simulink model "pdcm"  (R2019b)
settings: Solver=FixedStepAuto  StartTime=0.0  StopTime=10.0  FixedStep=0.1  RelTol=1e-3
settings Model: Creator=ADEMATO1  LastModifiedBy=EMORAI12
settings SolverCC: PositivePriorityOrder=on  AutoInsertRateTranBlk=on  InsertRTBMode=Always

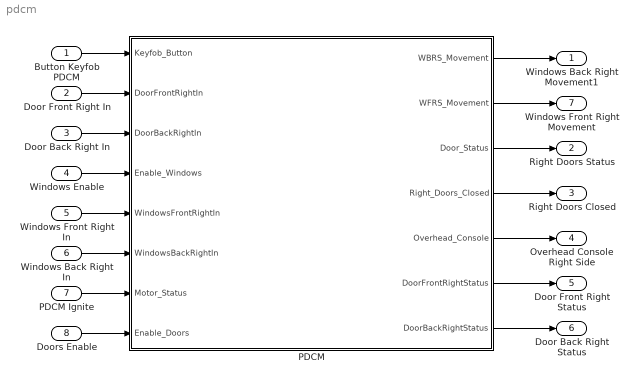
== system pdcm ==
  Button Keyfob PDCM : Inport
  Door Front Right In : Inport  Port=2
  Door Back Right In : Inport  Port=3
  Windows Enable : Inport  Port=4
  Windows Front Right In : Inport  Port=5
  Windows Back Right In : Inport  Port=6
  PDCM Ignite : Inport  Port=7
  Doors Enable : Inport  Port=8
  PDCM : Stateflow chart  TreatAsAtomicUnit=on
  Windows Back Right Movement1 : Outport
  Right Doors Status : Outport  Port=2
  Right Doors Closed : Outport  Port=3
  Overhead Console Right Side : Outport  Port=4
  Door Front Right Status : Outport  Port=5
  Door Back Right Status : Outport  Port=6
  Windows Front Right Movement : Outport  Port=7
  wires:
  PDCM/5(Overhead_Console) -> Overhead Console Right Side/1
  Windows Back Right In/1 -> PDCM/6(WindowsBackRightIn)
  PDCM/4(Right_Doors_Closed) -> Right Doors Closed/1
  Windows Front Right In/1 -> PDCM/5(WindowsFrontRightIn)
  Button Keyfob PDCM/1 -> PDCM/1(Keyfob_Button)
  Door Back Right In/1 -> PDCM/3(DoorBackRightIn)
  PDCM Ignite/1 -> PDCM/7(Motor_Status)
  Windows Enable/1 -> PDCM/4(Enable_Windows)
  Doors Enable/1 -> PDCM/8(Enable_Doors)
  Door Front Right In/1 -> PDCM/2(DoorFrontRightIn)
  PDCM/3(Door_Status) -> Right Doors Status/1
  PDCM/6(DoorFrontRightStatus) -> Door Front Right Status/1
  PDCM/7(DoorBackRightStatus) -> Door Back Right Status/1
  PDCM/1(WBRS_Movement) -> Windows Back Right Movement1/1
  PDCM/2(WFRS_Movement) -> Windows Front Right Movement/1

== stateflow chart pdcm/PDCM ==
  state Right_Doors_Enable
    state Right_Doors_Enable [parallel]
      during:
      if (Car_Unlocked == 1)
      DFRS = DoorFrontRightIn;
      DBRS = DoorBackRightIn;
      end
      if (DFRS == 1 | DBRS == 1)
      Overhead_Console = 1;
      Door_Status = 1;
      else
      Overhead_Console = 0;
      Door_Status = 0;
      end
      if (DFRS == 1)
      DoorFrontRightStatus = 1;
      else
      DoorFrontRightStatus = 0;
      end
      if (DBRS == 1)
      DoorBackRightStatus = 1;
      else
      DoorBackRightStatus = 0;
      end
      settings: executionOrder=1
    state Windows_Switch_When_TOff [parallel]
      during:
      if (aux2==1 &&  time ==1)
      WFRS_Movement = WindowsFrontRightIn;
      WBRS_Movement = WindowsBackRightIn;
      else
      WFRS_Movement = -1;
      WBRS_Movement = -1;
      end
      settings: executionOrder=2
    state count [parallel]
      settings: executionOrder=3
      state state_count
        entry :
        time =0;
        during :
        if(aux2==1)
        time =1;
        else
        time =0;
        end
      state state_count1
        during :
      (default) -> state_count
      state_count -> state_count1 : [time==1]
      state_count1 -> state_count : [after(10,sec)]{ aux2=0}
  state Wait_Car_On
    during:
    if(DFRS == 0 & DBRS == 0)
    Right_Doors_Closed = 1;
    end
    if(Enable_Windows == 0)
    WFRS_Movement = -1;
    WBRS_Movement = -1;
    end
    if (Enable_Windows == 1 && Enable_Doors == 1)
    AUX = 4 ;
    elseif  (Enable_Windows == 1)
    AUX = 1;
    elseif (Enable_Doors == 1)
    AUX = 3;
    else
    AUX = 2;
    end
  state State_Unlock_PDCM
    entry:
    Car_Unlocked = 1;
  state Lock_Unlock
    entry:
    Keyfob_Button;
    DFRS = 0;
    DBRS = 0;
    Door_Status = 0;
    WFRS_Movement = -1;
    WBRS_Movement = -1;
    Close_Windows = -1;
    aux2 = 0;
    AUX = 0;
  state Windows_Closed
    entry:
    WFRS_Movement = -1;
    WBRS_Movement = -1;
    Close_Windows = 0;
  state Windows_Update
  state state_transition
  state Windows_Control
    entry:
    aux1 = 0;
    WFRS = WindowsFrontRightIn;
    WBRS = WindowsBackRightIn;
    during:
    aux1 = 1;
    AUX = 2;
  state Right_Doors_Control
    entry:
    DFRS = DoorFrontRightIn;
    DBRS = DoorBackRightIn;
    during:
    if (DFRS == 1 | DBRS == 1)
    Overhead_Console = 1;
    Door_Status = 1;
    elseif (DFRS == 0 & DBRS == 0)
    Overhead_Console = 0;
    Door_Status = 0;
    end
    if (DFRS == 1)
    DoorFrontRightStatus = 1;
    else
    DoorFrontRightStatus = 0;
    end
    if (DBRS == 1)
    DoorBackRightStatus = 1;
    else
    DoorBackRightStatus = 0;
    end
    if (AUX ==3)
    AUX = 2;
    elseif (AUX==4)
    AUX=5;
    end
  state Closing_Windows
    entry:
    WFRS_Movement = 1;
    WBRS_Movement = 1;
  state State_Lock_PDCM
    entry:
    if (DFRS == 0 & DBRS == 0 & Keyfob_Button == 1 )
    Right_Doors_Closed = 1;
    Close_Windows = 1;
    Car_Unlocked = 0;
    else
    Close_Windows = 0;
    Right_Doors_Closed = 0;
    Car_Unlocked = 1;
    end
  State_Unlock_PDCM -> Right_Doors_Enable : [Enable_Doors == 1]
  State_Lock_PDCM -> Right_Doors_Enable [order 2] : [Car_Unlocked == 1 & Close_Windows == 0]
  Right_Doors_Enable -> State_Lock_PDCM [order 2] : [Keyfob_Button == 1]
  Right_Doors_Enable -> Wait_Car_On [order 1] : [Motor_Status == 1]
  Wait_Car_On -> Right_Doors_Enable [order 3] : [Motor_Status == 0]{aux2=1}
  (default) -> Lock_Unlock
  Lock_Unlock -> State_Unlock_PDCM [order 1] : [Keyfob_Button == 2]
  Windows_Update -> Wait_Car_On : after (200,msec)
  Windows_Closed -> State_Unlock_PDCM : [Keyfob_Button == 2]
  Lock_Unlock -> State_Lock_PDCM [order 2] : [Keyfob_Button == 1]
  Wait_Car_On -> Windows_Control [order 2] : [AUX == 1]
  Wait_Car_On -> Right_Doors_Control [order 1] : [AUX == 4 | AUX == 3]
  Right_Doors_Control -> Wait_Car_On [order 2] : [AUX == 2]
  (junction 227) -> state_transition [order 1] : [WFRS == 0] {WFRS_Movement = 0}
  Closing_Windows -> Windows_Closed : after(5,sec)
  state_transition -> Windows_Update [order 1] : [WBRS == -1] {WBRS_Movement = -1}
  state_transition -> Windows_Update [order 3] : [WBRS == 0] {WBRS_Movement = 0}
  state_transition -> Windows_Update [order 2] : [WBRS == 1] {WBRS_Movement = 1}
  Windows_Control -> (junction 227) : [aux1 == 1]
  (junction 227) -> state_transition [order 2] : [WFRS == -1] {WFRS_Movement = -1}
  (junction 227) -> state_transition [order 3] : [WFRS == 1] {WFRS_Movement = 1}
  Right_Doors_Control -> Windows_Control [order 1] : [AUX==5]
  (junction 220) -> Closing_Windows : after(3,sec)
  State_Lock_PDCM -> (junction 220) [order 1] : [Close_Windows == 1]
  data: enable_switches local; DWSdot local; BRWSdot local; BRWS local; PWS local; PWSdot local; BLWS local; BLWSdot local; DWS local; Keyfob_Button input; DoorFrontRightIn input; DoorBackRightIn input; Enable_Windows input; WindowsFrontRightIn input; WindowsBackRightIn input; Motor_Status input; WBRS_Movement output; WFRS_Movement output; Door_Status output; Right_Doors_Closed output; DFRS local; DBRS local; WFRS local; WBRS local; Overhead_Console output; Close_Windows local; next local; aux1 local; Enable_Doors input; AUX local; Car_Unlocked local; aux2 local; time local; DoorFrontRightStatus output; DoorBackRightStatus output
